simulink model "TrailerSoftware"  (R2019b)
settings: Solver=FixedStepDiscrete  StartTime=0.0  StopTime=inf  FixedStep=update  RelTol=1e-3  EnableMultiTasking=on
values from neighbouring files (symbols this model uses):
  countmax1 = 2500    [ProductionMfile.m]
  countmax2 = 2500    [ProductionMfile.m]
  HeaterIntGain = .0008    (= 0.0008)    [ProductionMfile.m]
  HeatGain = 10    [ProductionMfile.m]
  Intll = 0    [ProductionMfile.m]
  MaxCondPressure = 350    [ProductionMfile.m]
  MinSP = 1    [ProductionMfile.m]
  PostGain100 = 0.0002    [ProductionMfile.m]
  PostGain150 = 0.0005    [ProductionMfile.m]
  PostGain200 = 0.0004    [ProductionMfile.m]
  PostGain300 = 0.0008    [ProductionMfile.m]
  PostInit150 = 12    [ProductionMfile.m]
  PostIntulC = 65    [ProductionMfile.m]
  PostPGain = 0    [ProductionMfile.m]
  PreGain100 = 0.0005    [ProductionMfile.m]
  PreGain150 = 0.0005    [ProductionMfile.m]
  PreGain200 = 0.0003    [ProductionMfile.m]
  PreGain300 = 0.0008    [ProductionMfile.m]
  PreInit150 = 30    [ProductionMfile.m]
  PreIntulC = 65    [ProductionMfile.m]
  PreIntulDH = 65    [ProductionMfile.m]
  PrePGain = 0    [ProductionMfile.m]
  SatPress = [10 20 30 40 50 60 70 80 90 100 110 120 130 140 150 160 170      180 190 200 210 220 230 240 250 260 270 280 290 300 310 320 330      340 350 360 370 380 390 400 410 420 430 440 450 460 470 480 490      500]    [ProductionMfile.m]
  SatTemp = [-29.497 -2.4046 15.401 29.047 40.267 49.88 58.338 65.922 72.819      79.159 85.037 90.526 95.68 100.55 105.16 109.54 113.73 117.73 121.57      125.26 128.82 132.25 135.56 138.77 141.88 144.89 147.82 150.67 153.44      156.15 158.78 161.35 163.85 166.3 168.7 171.04 173.33 175.58 177.77      179.93 182.04 184.11 186.14 188.14 190.09 192.01 193.9 195.75 197.58      199.37]    [ProductionMfile.m]
  SHGain = 2    [ProductionMfile.m]
  SizeCANMatrix = 80    [ProductionMfile.m]
  SizeCOBIDVector = 10    [ProductionMfile.m]
  update = 0.002    [ProductionMfile.m]
undefined symbols (not defined in the file or in its folder): DiscIntNeverNeededParam, PostDGain, PreDGain, Ratio100, Ratio150, Ratio200, Ratio300
libraries: simulink x60, c2837xDlib x35, xpcutilitieslib x24, c2802xlib x8, c280xlib x7, etargetslib x4, svdutilitieslib x2, c2000lib x1
(part 5 of 8)

== stateflow chart TrailerSoftware/SPI Interface/Chart ==
  state Master1
    state Step1
      entry:
      StateNum = 1;
      Ready1 = CheckReady1;
      if GoToMaster == uint16(1);
      GoToTemps= uint16(0);
      else
      GoToTemps = uint16(1);
      end
    state Step2
      entry:
      StateNum = 2;
      if GoToMaster == uint16(1);
      GoToAuxGPIO = uint16(0);
      else
      GoToAuxGPIO = uint16(1);
      end
    state Step3
      entry:
      StateNum = 3;
      if GoToMaster == uint16(1);
      GoToDisplay = uint16(0);
      else
      GoToDisplay = uint16(1);
      end
    state Ready = CheckReady1 [function]
    (default) -> Master1.Step1
    Master1.Step1 -> Master1.Step2 [order 2] : [GoToTemps == uint16(0)]{GoToMaster = uint16(0);}
    Step3 -> Master1.Step1 [order 1] : [GoToDisplay == uint16(0)]{GoToMaster = uint16(0);}
    Master1.Step2 -> Step3 [order 1] : [GoToAuxGPIO == uint16(0)]
        | {GoToMaster = uint16(0);}
  state Display
    state Step1
      entry:
      StateNum = 8;
      GoToMaster = 1;
      DisplayInitComplete = 1;
      GoToDisplay = 0;
    (default) -> Display.Step1
  state AuxGPIO
    state Step1
      entry:
      StateNum = 6;
      GoToAuxGPIO = uint16(0);
      CSLow;
      Write;
      Address(uint16(10)); % Write to ICON
      Data(uint16(8));
      CSHigh
      CSLow;
      Write;
      Address(uint16(0)); % Write to IODIRA
      Data(uint16(0));
      CSHigh
      CSLow;
      Write;
      Address(uint16(1)); % Write to ODIRB
      Data(uint16(255));
      CSHigh
      AuxInitGPIO = uint16(1);
    state CSLow [function]
    state CSHigh [function]
    state Step2
      entry:
      StateNum = 7;
      CSLow;
      Write;
      Address(uint16(18)); % GPIOA Write to outputs
      Data(AuxGPIOOutput);
      CSHigh
      CSLow
      Read;
      Address(uint16(19));  % Read from inputs GPIOB
      AuxGPIOInput = Output;
      CSHigh
      GoToMaster = uint16(1);
    (default) -> AuxGPIO.Step1
    AuxGPIO.Step1 -> AuxGPIO.Step2
  state Temps
    state CSLowTemp1 [function]
    state Step1
      entry:
      StateNum = 4;
      value = uint16(0);
      fault = uint16(0);
      GoToMaster = uint16(0);
      CSLowTemp1;
      Address(uint16(128));
      value = Data(uint16(66));
      CSHighTemp1;
      CSLowTemp1;
      Address(uint16(7));
      fault = Data(uint16(0));
      CSHighTemp1;
      TempsInitComplete = uint16(1);
      GoToMaster = uint16(1);
    state CSHighTemp1 [function]
    state Step2
      entry:
      StateNum = 5;
      GoToMaster = uint16(0);
      CSLowTemp1;
      Address(uint16(1));
      MSB = Data(uint16(0));
      CSHighTemp1;
      CSLowTemp1;
      Address(uint16(2));
      LSB = Data(uint16(0));
      CSHighTemp1;
      [TOut1,TFault1] = TempCal(MSB,LSB);
      GoToMaster = uint16(1);
    state [TOut,TFault] = TempCal(MSB,LSB) [function]
    Temps.Step2 -> (junction 214) : [GoToMaster == uint16(1) ]
    Temps.Step1 -> (junction 214) : [GoToMaster == uint16(1) ]
  state Read [function]
  state Out1 = Data(value) [function]
  state Write [function]
  state Address(value) [function]
  state Contents = Output [function]
  Master1.Step1 -> Temps.Step2 [order 3] : [(GoToTemps == uint16(1) ) &&...
      |   (TempsInitComplete == uint16(1))]
  Master1.Step2 -> AuxGPIO.Step1 [order 3] : [GoToAuxGPIO == uint16(1) && ...
      | AuxInitGPIO == uint16(0)]
  (junction 214) -> Master1.Step1 : [(GoToTemps == uint16(1) ) && ...
      |  (TempsInitComplete == uint16(1))]
  (default) -> Master1
  Master1.Step2 -> AuxGPIO.Step2 [order 2] : [GoToAuxGPIO == uint16(1) && ...
      | AuxInitGPIO == uint16(1)]
  Step3 -> Display.Step1 [order 2] : [GoToDisplay == uint16(1)]
  Master1.Step1 -> Temps.Step1 [order 1] : [(GoToTemps == uint16(1)) &&...
      |  (TempsInitComplete == uint16(0))]
  AuxGPIO.Step2 -> Master1.Step2 : [GoToMaster == uint16(1)]
  Display.Step1 -> Step3 : [GoToMaster == uint16(1)]
  data: Ready function_output size=1; MSB function_input uint16 size=1; LSB function_input uint16 size=1; TOut function_output uint16 size=1; TFault function_output uint16 size=1; value function_input uint16 size=1; Out1 function_output uint16 size=1; value function_input uint16 size=1; Contents function_output uint16; GoToDisplay local uint16 size=1 =uint16(0); GoToAuxGPIO local uint16 size=1 =uint16(0); GoToMaster local uint16 size=1 =uint16(0); GoToTemps local uint16 size=1 =uint16(0); DisplayInitComplete local uint16 size=1 =uint16(0); AuxGPIOOutput input uint16 size=1; AuxGPIOInput output uint16; AuxInitGPIO local; value output; TFault1 output; fault local; TOut1 output; Ready1 local uint16 size=1; StateNum output uint16 size=1; LSB output; MSB output; TempsInitComplete output uint16 size=1 =uint16(0)

== matlab function TrailerSoftware/Subsystem/Display ==
  data: DisRow1 output; DisRow2 output; DisRow3 output; DisRow4 output; StartRow1 output; StartRow2 output; StartRow3 output; StartRow4 output; NumCharRow1 output; NumCharRow2 output; NumCharRow3 output; NumCharRow4 output; ClearDisplay output; DisplayDataAvail output; time input; MBV input; HeaterTempCom input; UseHeater input; CoolTempCom input; PressCommand input; warning1 input; warning2 input; warning3 input; fault1 input; fault2 input; fault3 input; Pulse input; FlowRate input; DuctTemp input; DuctPress input; DuctTempIn input; Hin input; Hout input
function [DisRow1,DisRow2,DisRow3,DisRow4,StartRow1,StartRow2,...
    StartRow3,StartRow4,NumCharRow1,NumCharRow2,NumCharRow3,NumCharRow4,...
    ClearDisplay,DisplayDataAvail]= fcn(time,MBV,...
    HeaterTempCom,UseHeater,CoolTempCom,PressCommand,warning1,warning2,warning3,fault1,fault2,...
    fault3,Pulse,FlowRate,DuctTemp,DuctPress,DuctTempIn,Hin,Hout)
persistent time0 count1 count2 displ  
if isempty(time0)
    time0 = time;
    count1 = 1;
    count2 = 1;
    displ = 0;
end
DisplayDataAvail = 0; %#ok<*NASGU>
if Pulse == 1
    DisplayDataAvail = 1;
end

TempCommand = CoolTempCom;
if UseHeater == 1
    TempCommand = HeaterTempCom;  
end
%#codegen
% MBV(1) = SystemStateValue;
%   Value  Name     Description 
%   0x0090 Menu     Controller is in the menu system
%   0x0093 Off      Controller is in the off mode
%   0x0096 Auto     Controller is in the auto mode
%   0x0099 Failure  Controller is in the failure mode
%   0x009C Running  Controller is in the running mode
% MBV(2) = RunningStateValue;
%   Value  Index        Name               Description
%   0x00   1            No Running         Mode Controller is not in any running state
%   0x01   2            Delay to Start     Controller is delaying to start
%   0x02   3            Preheat            Controller is preheating engine
%   0x03   4            Cranking           Controller is cranking engine
%   0x04   5            Crank Rest         Controller is resting before next crank
%   0x05   6            Crank Success      Controller has successfully started engine
%   0x06   7            Reserved           Reserved
%   0x07   8            Warmup             Controller is warming up engine before applying load
%   0x08   9            Running            Controller is in a normal running state
%   0x09   10           Cooldown           Controller is cooling down engine before shutting down
%   0x0A   11           Shutdown           Controller has shut down the engine
%   0x0B   12           Failure            Controller has shut down the engine due to a fault
%   0x20   13           Remote             Controller was started from 'Start / Stop' switched input
%   0x21   14           Manual             Controller was started from the front panel button
%   0x22   15           Modbus             Controller was started by Modbus command
%   0x23   16           Battery Recharge   Controller was started to recharge batteries
%   0x24   17           Exerciser          Controller was started from the exerciser clock
%   0x25   18           Auxiliary Sensor 1 Controller was started based on Auxiliary Sensor 1 reading
%   0x26   19           Auxiliary Sensor 2 Controller was started based on Auxiliary Sensor 2 reading
%   0x27   20           Loss of Mains      Controller was started due to loss of mains voltage
%   0x28   21           Momentary Switch   Controller was started from 'Momentary' switched input
%   0x29   22           Auxiliary Sensor 3 Controller was started based on Auxiliary Sensor 3 reading
%   0x2A   23           Auxiliary Sensor 4 Controller was started based on Auxiliary Sensor 4 reading
%    RunningState = MBV(2) + 1;


% MBV(3) = EventBitMap1ValueA;
%   Value  Description
%   0      Not In Auto Bit is on due to controller not being in auto mode
%   1      Idle Mode Bit is on due to controller being in idle mode
%   2      Battle Mode Bit is on due to controller being in battle mode
%   3      System OK Bit is on due to controller being free of warnings and failures
%   4      Glowplug Bit is on due to 'Preheat' timer
%   5      Warmup Bit is on due to 'Warmup' timer
%   6      Cooldown Bit is on due to 'Cooldown' timer
%   7      Engine Running Bit is on due to engine running
%   8      Exerciser Bit is on due to engine exercise
%   9      Battery Recharge Bit is on due to battery recharge
%   10     Maintenance Required Bit is on due to 'Maintenance Counter' timer expiring
%   11     Low Battery During Cranking Bit is on due to 'Low Battery Voltage During Cranking'
%   12     N/A
%   13     N/A
%   14     N/A
%   15     N/A 
    
% MBV(4) = EventBitMap1ValueB;
%   0      Delay to Start Bit is on due to 'Delay to Start' timer
%   1      Force Regeneration Bit is on due to a force regeneration (DPF)
%   2      Regeneration Inhibit Bit is on due to regeneration being inhibited (DPF)
%   3 ~ 7  Reserved Reserved
%   8      Fuel Bit is on due to fuel output enabled
%   9      Crank Bit is on due to crank output enabled
%   10     Genset Break1 Bit is on due to transferring to generator position
%   11     Mains Break1 Bit is on due to transferring to mains position
%   12     Pull Coil Bit is on due to pull coil being enabled
%   13     LCD Backlight Bit is on due to the LCD backlight being on
%   14     Voltage Regulator Bit is on when controller is not in idle mode
%   15     Energize to Stop Bit is on due to Energize to Stop timer
% MBV(5) = EventBitMap2ValueA;
%   0      Group Output 1 Bit is on due to output set to Group Output 1 is active
%   1      Group Output 2 Bit is on due to output set to Group Output 2 is active
%   2      Group Output 3 Bit is on due to output set to Group Output 3 is active
%   3      Group Output 4 Bit is on due to output set to Group Output 4 is active
%   4      Increment RPM Bit is on due to the RPM being manually incremented through speed
%          control
%   5      Decrement RPM Bit is on due to the RPM being manually decremented through speed
%          control
%   6      DEF Fluid Pump Bit is on due to DEF Fluid Pump being on
%   7      Genset Disable Bit is on due to the Genset being disabled
%   8      Dummy Load ON Bit is on due to Dummy Load being enabled
%   9 ~ 11 Reserved Reserved
%   12     Glowplug Bit is on due to preheat input or ECM preheat being active
%   13     Common Fault Bit is on due to a any fault occurring
%   14     Temperature Unit Reserved - Fixed to Fahrenheit
%   15     Pressure Unit Reserved - Fixed to PSI
% MBV(6) = EventBitMap2ValueB;
%   0      Overcrank Warning Bit is on due to controller failing to crank engine on first attempt
%   1      Invalid Setting Warning Bit is on due to an invalid setting being stored in the controller
%   2      Emergency Input Bit is on due to Emergency Stop input being active
%   3      EPS Load is On Bit is on due to current readings being at least 5% of the rated current
%          setting
%   4      Genset Break On1 Reserved
%   5      Mains Break On1 Reserved
%   6      Mains Pickup1 Bit is on due to mains voltage being within acceptable levels after
%          dropping out
%   7      Mains Dropout1 Bit is on due to controller sensing mains voltage has dropped out
%   8      Mains OK1 Bit is on due to mains voltage being within acceptable levels
%   9      Start Inhibit Bit is on due to Start Inhibit input being active
%   10     Remote Reset Bit is on due to the Remote Reset input being active
%   11 ~15 N/A
% MBV(7) = FaultBitMapValueA;
%   Bit   Name                  Description
%   0     Overcrank             Fault due to max attempts at cranking
%   without starting (1)
%   1     Engine Failed to Stop Fault due to engine speed not being 0 RPM
%   at shutdown (2)
%   2     DM1 Stop Lamp1        DM1 Stop Lamp is on (not used) (3)
%   3     High Engine Temp      Fault due to high engine temperature (4)
%   4     Low Oil Pressure      Fault due to low oil pressure (5)
%   5     Low Fuel Level        Fault due to low fuel level (6)
%   6     Under Speed           Fault due to low engine speed (7)
%   7     Over Speed            Fault due to high engine speed (8)
%   8     Low Battery Voltage   Fault due to low battery voltage (9)
%   9     High Battery Voltage  Fault due to high battery voltage (10)
%   10    Low Coolant Level     Fault due to low coolant level (11)
%   11    Low Air Pressure      Fault due to low air pressure (not used)
%   (12)
%   12    Low Hydraulic Press   Fault due to low hydraulic pressure (not
%   used) (13)
%   13    Under Frequency       Fault due to low AC frequency (14)
%   14    Over Frequency        Fault due to high AC frequency (15)
%   15    AC Under Voltage      Fault due to low AC voltage (16)
% MBV(8) = FaultBitMapValueB;
%   0     AC Over Voltage       Fault due to high AC voltage (17)
%   1     ECM Communication     Fault due to loss of communications with
%   ECM (18)
%   2     Configurable Failure 1 Fault due to Configurable Fail Input 1
%   being active (not used) (19)
%   3     Configurable Failure 2 Fault due to Configurable Fail Input 2
%   being active (not used) (20)
%   4     Auxiliary Sensor 1    Fault due to low / high reading on
%   Auxiliary Sensor 1  (not used) (21)
%   5     Auxiliary Sensor 2    Fault due to low / high reading on
%   Auxiliary Sensor 2 (not used) (22)
%   6     Auxiliary Sensor 3    Fault due to low / high reading on Auxiliary Sensor 3 
%   (not used) (23)
%   7     Auxiliary Sensor 4    Fault due to low / high reading on
%   Auxiliary Sensor 4 (not used) (24)
%   8     Over Current          Fault due to high current reading (25)
%   9     Configurable Failure 3 Fault due to Configurable Fail Input 3
%   being active (not used) (26)
%   26 ~ 31 Reserved Reserved (not used) (27-32)
       
%   Bit   Name                  Description
%   0     Low Engine Temp       Warning due to low engine temperature
%   1     High Engine Temp      Warning due to high engine temperature
%   2     Low Oil Pressure      Warning due to low oil pressure
%   3     Under Speed           Warning due to low engine speed
%   4     Over Speed            Warning due to high engine speed
%   5     Low Fuel Level        Warning due to low fuel level
%   6     High Fuel Level       Warning due to high fuel level
%   7     Low Battery Voltage   Warning due to low battery voltage
%   8     High Battery Voltage  Warning due to high battery voltage
%   9     Under Frequency       Warning due to low AC frequency
%   10    Over Frequency        Warning due to high AC frequency
%   11    AC Under Voltage      Warning due to low AC voltage
%   12    AC Over Voltage       Warning due to high AC voltage
%   13    Battery Charger Fault Warning due to battery charger fault
%   14    Over Current          Warning due to high AC current
%   15    Fuel In Basin         Warning due to fuel being in the catch basin
% MBV(10) = WarningBitMapValueB;
%   Bit   Name                  Description
%   0     Configurable Warning 1 Warning due to Configurable Warn Input 1 being active
%   1     Configurable Warning 2 Warning due to Configurable Warn Input 2 being active
%   2     Auxiliary Sensor 1     Warning due to low / high reading on Auxiliary Sensor 1
%   3     Auxiliary Sensor 2     Warning due to low / high reading on Auxiliary Sensor 2
%   4     Auxiliary Sensor 3     Warning due to low / high reading on Auxiliary Sensor 3
%   5     Auxiliary Sensor 4     Warning due to low / high reading on Auxiliary Sensor 4
%   6 ~ 15 Reserved Reserved
% MBV(11) = GenFreqValue;
% MBV(12) = GenVoltValueA;
% MBV(13) = GenVoltValueB;
% MBV(14) = GenVoltValueC;
% MBV(15) = GenCurValueA;
% MBV(16) = GenCurValueB;
% MBV(17) = GenCurValueC;
% MBV(18) = EngineTempValue;
% MBV(19) = EngineOilPressValue;
% MBV(20) = FuelLevelValue;
% MBV(21) = BatteryVoltValue;
% MBV(22) = EngineRunHoursValue;
% MBV(23) = FCSuperHeatValue;
% MBV(24) = RCSuperHeatValue;
% MBV(25) = SuctionPressValue;
% MBV(26) = FSatTempValue;
% MBV(27) = RSatTempValue;
% MBV(28) = FSucTempValue;
% MBV(29) = RSucTempValue;
% MBV(30) = FRmTempValue;
% MBV(31) = RRmTempValue;
% MBV(32) = FValPosValue;
% MBV(33) = RValPosValue;
% MBV(34) = FEvapTempValue;
% MBV(35) = REvapTempValue;
% MBV(36) = FAlarmValue;
% MBV(37) = RAlarmValue;

FuelLevelValue = MBV(20);
s1 = convertnum(FuelLevelValue);
s2 = convertnum(FlowRate);
s6 = convertnum(min(140,max(TempCommand,0)));
s7 = convertnum(min(9,max(PressCommand,0)));
s8 = convertnum(min(140,max(DuctTemp,0)));
s9 = convertnum(min(9,max(DuctPress,0)));
s10 = convertnum(min(140,max(DuctTempIn,0)));
s11 = convertnum(min(99,max(Hin,0)));
s12 = convertnum(min(99,max(Hout,0)));
Message1 = ['TempSet ' s6(1:3)...
    ',Meas' s8(1:3) 'F'];
Message2 = ['PSet' s7(1:4)...
    ',Meas' s9(1:4) 'psi'];
Message3 = ['Inlet Air Temp: ' s10...
    ', deg F  ','Fuel Level ' s1...
    ',% ' 'Humidity Inlet ' s11...
    ',% ' 'Humidity Outlet ' s12...
    ',% '  'Flow Rate Selected = ' s2...
    ', lbm/min'];
    
s4A = convertnum(min(999,max(warning1,0)));
s4B = convertnum(min(999,max(warning2,0)));
s4C = convertnum(min(999,max(warning3,0)));
s5A = convertnum(min(999,max(fault1,0)));
s5B = convertnum(min(999,max(fault2,0)));
s5C = convertnum(min(999,max(fault3,0)));

 Message4 = [' Warning = ' s4A ' ' s4B ' ' s4C ' Fault = ' s5A...
        ' ' s5B ' ' s5C ' '];

DisRow1 = uint8(32*ones(20,1));
DisRow2 = uint8(32*ones(20,1));
DisRow3 = uint8(32*ones(20,1));
DisRow4 = uint8(32*ones(20,1));
StartRow1 = uint8(1);
StartRow2 = uint8(1);
StartRow3 = uint8(1);
StartRow4 = uint8(1);
NumCharRow1 = uint8(20);
NumCharRow2 = uint8(20);
NumCharRow3 = uint8(20);
NumCharRow4 = uint8(20);
ClearDisplay = uint8(0);
DisplayDataAvail = uint8(0);
if displ == 1
    DisplayDataAvail = uint8(1);
    displ = 0;
end
if time > time0 + .5
    time0 = time;
    displ = 1;
    count1 = count1 + 1;
    count2 = count2 + 1;
    if count1 == length(Message3) - 20
        count1 = 1;
    end
    if count2 == length(Message4) - 20
        count2 = 1;
    end
end
    
DisRow1(:,1) = Message1;
DisRow2(:,1) = Message2;
DisRow3(:,1) = Message3(1,count1:count1+19)';
DisRow4(:,1) = Message4(1,count2:count2+19)';

return

% Convert number to string
function y = convertnum(input)
    y = uint8(32*ones(1,5));
    int_part = double(floor(input));
    float_part = input - double(int_part);
    i = 1;
    temp = int_part;
    if temp < 10
        y(i) = uint8(temp + 48);  
        i = 2;
    elseif floor(temp/10) < 10
        y(i) = uint8(floor(temp/10)+48);
        y(i+1) = uint8((temp - floor(temp/10)*10) + 48);
        i = 3;
    elseif floor(temp/100) < 10
        y(i) = uint8(floor(temp/100)+48);
        y(i+1) = uint8(floor((temp - floor(temp/100)*100)/10) + 48);
        y(i+2) = uint8((temp - floor(temp/10)*10) + 48);
        i = 4;
    end
    y(i) = '.';
    temp = float_part;
    i = i + 1;
    if temp*10 < 10
        y(i) = uint8((temp*10) + 48);  
    end
    
return

== matlab function TrailerSoftware/Subsystem/Modbus Routine ==
  data: ModbusInputReady input uint8; ModbusOutReady output uint8; ModbusInputVector input; ModbusOutVector output size=[1,8]; time input; ModbusVector output size=39; countoutputout output; ManualMode2StatusOut output size=1; ManualMode3StatusOut output size=1; Failcountout output; Goodcountout output; FaultBitMapValueAOut output
function [ModbusOutReady,ModbusOutVector,ModbusVector,...
    countoutputout,ManualMode2StatusOut,...
    ManualMode3StatusOut,Failcountout,Goodcountout,...
    FaultBitMapValueAOut] = fcn1(ModbusInputReady,ModbusInputVector,time)
persistent SystemState RunningState EventBitMap1A EventBitMap1B ...
    EventBitMap2A EventBitMap2B FaultBitMapA FaultBitMapB WarningBitMapA ...
    WarningBitMapB GenFreq GenVoltA GenVoltB GenVoltC GenCurA GenCurB ...
    GenCurC EngineTemp EngineOilPress FuelLevel EngineRunHours....
    BatteryVolt State time0 SystemStateValue ...
    RunningStateValue EventBitMap1ValueA  EventBitMap1ValueB ...
    EventBitMap2ValueA EventBitMap2ValueB FaultBitMapValueA ...
    FaultBitMapValueB WarningBitMapValueA WarningBitMapValueB ...
    GenFreqValue GenVoltValueA GenVoltValueB GenVoltValueC ...
    GenCurValueA GenCurValueB GenCurValueC EngineTempValue ...
    EngineOilPressValue FuelLevelValue BatteryVoltValue ...
    EngineRunHoursValue  countinput...
    countoutput ManualMode2Status...
    ManualMode3Status complete Failcount Goodcount SuctionOutCnt...
    SuctionInCnt Goodcount1300
if isempty(SystemState)
    
    SystemState = [hex2dec('01') hex2dec('03') hex2dec('00')...
                hex2dec('A7') hex2dec('00') hex2dec('01')...
                hex2dec('35') hex2dec('E9')];
    RunningState = [hex2dec('01') hex2dec('03') hex2dec('00')...
                hex2dec('A8') hex2dec('00') hex2dec('01')...
                hex2dec('05') hex2dec('EA')];
    EventBitMap1A = [hex2dec('01') hex2dec('03') hex2dec('00')...
                hex2dec('B6') hex2dec('00') hex2dec('01')...
                hex2dec('65') hex2dec('EC')];
    EventBitMap1B = [hex2dec('01') hex2dec('03') hex2dec('00')...
                hex2dec('B7') hex2dec('00') hex2dec('01')...
                hex2dec('34') hex2dec('2C')];    
    EventBitMap2A = [hex2dec('01') hex2dec('03') hex2dec('00')...
                hex2dec('B8') hex2dec('00') hex2dec('01')...
                hex2dec('04') hex2dec('2F')];
    EventBitMap2B = [hex2dec('01') hex2dec('03') hex2dec('00')...
                hex2dec('B7') hex2dec('00') hex2dec('01')...
                hex2dec('34') hex2dec('2C')];
    FaultBitMapA = [hex2dec('01') hex2dec('03') hex2dec('00')...
                hex2dec('B5') hex2dec('00') hex2dec('01')...
                hex2dec('95') hex2dec('EC')];
    FaultBitMapB = [hex2dec('01') hex2dec('03') hex2dec('00')...
                hex2dec('B6') hex2dec('00') hex2dec('01')...
                hex2dec('65') hex2dec('EC')];
    WarningBitMapA = [hex2dec('01') hex2dec('03') hex2dec('00')...
                hex2dec('B2') hex2dec('00') hex2dec('01')...
                hex2dec('24') hex2dec('2D')];
    WarningBitMapB = [hex2dec('01') hex2dec('03') hex2dec('00')...
                hex2dec('B3') hex2dec('00') hex2dec('01')...
                hex2dec('75') hex2dec('ED')];
    GenFreq = [hex2dec('01') hex2dec('03') hex2dec('00')...
                hex2dec('99') hex2dec('00') hex2dec('01')...
                hex2dec('54') hex2dec('25')];
    GenVoltA = [hex2dec('01') hex2dec('03') hex2dec('00')...
                hex2dec('9B') hex2dec('00') hex2dec('01')...
                hex2dec('F5') hex2dec('E5')];
    GenVoltB = [hex2dec('01') hex2dec('03') hex2dec('00')...
                hex2dec('9C') hex2dec('00') hex2dec('01')...
                hex2dec('44') hex2dec('24')];
    GenVoltC = [hex2dec('01') hex2dec('03') hex2dec('00')...
                hex2dec('9D') hex2dec('00') hex2dec('01')...
                hex2dec('15') hex2dec('E4')];
    GenCurA = [hex2dec('01') hex2dec('03') hex2dec('00')...
                hex2dec('9E') hex2dec('00') hex2dec('01')...
                hex2dec('E5') hex2dec('E4')];
    GenCurB = [hex2dec('01') hex2dec('03') hex2dec('00')...
                hex2dec('9F') hex2dec('00') hex2dec('01')...
                hex2dec('B4') hex2dec('24')];
    GenCurC = [hex2dec('01') hex2dec('03') hex2dec('00')...
                hex2dec('A0') hex2dec('00') hex2dec('01')...
                hex2dec('84') hex2dec('28')];
    EngineTemp = [hex2dec('01') hex2dec('03') hex2dec('00')...
                hex2dec('96') hex2dec('00') hex2dec('01')...
                hex2dec('64') hex2dec('26')];
    EngineOilPress = [hex2dec('01') hex2dec('03') hex2dec('00')...
                hex2dec('97') hex2dec('00') hex2dec('01')...
                hex2dec('35') hex2dec('E6')];
    FuelLevel = [hex2dec('01') hex2dec('03') hex2dec('00')...
                hex2dec('98') hex2dec('00') hex2dec('01')...
                hex2dec('05') hex2dec('E5')];
    BatteryVolt = [hex2dec('01') hex2dec('03') hex2dec('00')...
                hex2dec('9A') hex2dec('00') hex2dec('01')...
                hex2dec('A4') hex2dec('25')];
    EngineRunHours = [hex2dec('01') hex2dec('03') hex2dec('00')...
                hex2dec('A3') hex2dec('00') hex2dec('01')...
                hex2dec('74') hex2dec('28')];
    Goodcount1300 = 0;        
    State = 0;
    time0 = time;
    SystemStateValue = 0;
    RunningStateValue = 0;
    EventBitMap1ValueA = 0;
    EventBitMap1ValueB = 0;
    EventBitMap2ValueA = 0;
    EventBitMap2ValueB = 0;
    FaultBitMapValueA = 0;
    FaultBitMapValueB = 0;
    WarningBitMapValueA = 0;
    WarningBitMapValueB = 0;
    GenFreqValue = 0;
    GenVoltValueA = 0;
    GenVoltValueB = 0;
    GenVoltValueC = 0;
    GenCurValueA = 0;
    GenCurValueB = 0;
    GenCurValueC = 0;
    EngineTempValue = 0;
    EngineOilPressValue = 0;
    FuelLevelValue = 0;
    BatteryVoltValue = 0;
    EngineRunHoursValue = 0;
    countinput = 0;
    countoutput = 0;
    ManualMode2Status = 0;
    ManualMode3Status = 0;
    complete = 1;
    Failcount = 0;
    Goodcount = 0;
    SuctionOutCnt = 0;
    SuctionInCnt = 0;
end
%#codegen
if ModbusInputReady == 1
    countinput = countinput + 1;
end
countinputout = countinput;
ModbusOutReady = 0;
ModbusOutVector = SystemState;
%waittime1 = .75;
%waittime2 = 1.5;
%waittime3 = .01;
%waittime4 = .01;
timeout = 2;
ModbusVector = zeros(39,1);
countoutputout =  countoutput;
ManualMode2StatusOut = uint8(ManualMode2Status);
ManualMode3StatusOut = uint8(ManualMode3Status);
AutoMode =  double(not((bitget(uint32(EventBitMap1ValueA),1))));
Failcountout = Failcount;
Goodcountout = Goodcount;
SuctionOutCntOut = SuctionOutCnt;
SuctionInCntOut = SuctionInCnt;
Goodcount1300Out = Goodcount1300;
FaultBitMapValueAOut=FaultBitMapValueA;
switch State
    case 0
        ModbusOutVector = SystemState;
        ModbusOutReady = 1;
        State = 100;
        time0 = time;
    case 100
       if complete == 1
            State = 200;
            complete = 0;
       end
       if (time-time0) > timeout
            State = 200;
            complete = 0;
            Failcount = Failcount + 1;
       end 
    case 200
        ModbusOutVector = RunningState;
        ModbusOutReady = 1;
        State = 300;
        time0 = time;
    case 300
        if complete == 1
            State = 400;
            complete = 0;
        end
        if (time-time0) > timeout
            State = 400;
            complete = 0;
            Failcount = Failcount + 1;
       end 
    case 400
        ModbusOutVector = EventBitMap1A;
        ModbusOutReady = 1;
        State = 500;
        time0 = time;
    case 500
        if complete == 1
            State = 600;
            complete = 0;
        end
        if (time-time0) > timeout
            State = 600;
            complete = 0;
            Failcount = Failcount + 1;
       end 
    case 600
        ModbusOutVector = EventBitMap1B;
        ModbusOutReady = 1;
        State = 700;
        time0 = time;
    case 700
        if complete == 1
            State = 800;
            complete = 0;
        end
        if (time-time0) > timeout
            State = 800;
            complete = 0;
            Failcount = Failcount + 1;
        end 
    case 800
        ModbusOutVector = EventBitMap2A;
        ModbusOutReady = 1;
        State = 900;
        time0 = time;
    case 900
        if complete == 1
            State = 1000;
            complete = 0;
        end
        if (time-time0) > timeout
            State = 1000;
            complete = 0;
            Failcount = Failcount + 1;
       end 
    case 1000
        ModbusOutVector = EventBitMap2B;
        ModbusOutReady = 1;
        State = 1100;
        time0 = time;
    case 1100
        if complete == 1
            State = 1200;
            complete = 0;
        end
        if (time-time0) > timeout
            State = 1200;
            complete = 0;
            Failcount = Failcount + 1;
       end 
    case 1200
        ModbusOutVector = FaultBitMapA;
        ModbusOutReady = 1;
        State = 1300;
        time0 = time;
    case 1300
        if complete == 1
            State = 1400;
            complete = 0;
        end
        if (time-time0) > timeout
            State = 1400;
            complete = 0;
            Failcount = Failcount + 1;
       end 
    case 1400
        ModbusOutVector = FaultBitMapB;
        ModbusOutReady = 1;
        State = 1500;
        time0 = time;
    case 1500
        if complete == 1
            State = 1600;
            complete = 0;
        end
        if (time-time0) > timeout
            State = 1600;
            complete = 0;
            Failcount = Failcount + 1;
       end 
    case 1600
        ModbusOutVector = WarningBitMapA;
        ModbusOutReady = 1;
        State = 1700;
        time0 = time;
    case 1700
        if complete == 1
            State = 1800;
            complete = 0;
        end
        if (time-time0) > timeout
            State = 1800;
            complete = 0;
            Failcount = Failcount + 1;
       end 
    case 1800
        ModbusOutVector = WarningBitMapB;
        ModbusOutReady = 1;
        State = 1900;
        time0 = time;
    case 1900
        if complete == 1
            State = 2000;
            complete = 0;
        end
        if (time-time0) > timeout
            State = 2000;
            complete = 0;
            Failcount = Failcount + 1;
       end 
    case 2000
        ModbusOutVector = GenFreq;
        ModbusOutReady = 1;
        State = 2100;
        time0 = time;
    case 2100
         if complete == 1
            State = 2200;
            complete = 0;
        end
        if (time-time0) > timeout
            State = 2200;
            complete = 0;
            Failcount = Failcount + 1;
       end 
    case 2200
        ModbusOutVector = GenVoltA;
        ModbusOutReady = 1;
        State = 2300;
        time0 = time;
    case 2300
        if complete == 1
            State = 2400;
            complete = 0;
        end
        if (time-time0) > timeout
            State = 2400;
            complete = 0;
            Failcount = Failcount + 1;
       end 
    case 2400
        ModbusOutVector = GenVoltB;
        ModbusOutReady = 1;
        State = 2500;
        time0 = time;
    case 2500
        if complete == 1
            State = 2600;
            complete = 0;
        end
        if (time-time0) > timeout
            State = 2600;
            complete = 0;
            Failcount = Failcount + 1;
       end 
    case 2600
        ModbusOutVector = GenVoltC;
        ModbusOutReady = 1;
        State = 2700;
        time0 = time;
    case 2700
        if complete == 1
            State = 2800;
            complete = 0;
        end
        if (time-time0) > timeout
            State = 2800;
            complete = 0;
            Failcount = Failcount + 1;
       end 
    case 2800
        ModbusOutVector = GenCurA;
        ModbusOutReady = 1;
        State = 2900;
        time0 = time;
    case 2900
        if complete == 1
            State = 3000;
            complete = 0;
        end
        if (time-time0) > timeout
            State = 3000;
            complete = 0;
            Failcount = Failcount + 1;
       end 
    case 3000
        ModbusOutVector = GenCurB;
        ModbusOutReady = 1;
        State = 3100;
        time0 = time;
    case 3100
        if complete == 1
            State = 3200;
            complete = 0;
        end
        if (time-time0) > timeout
            State = 3200;
            complete = 0;
            Failcount = Failcount + 1;
       end 
    case 3200
        ModbusOutVector = GenCurC;
        ModbusOutReady = 1;
        State = 3300;
        time0 = time;
    case 3300   
        if complete == 1
            State = 3400;
            complete = 0;
        end
        if (time-time0) > timeout
            State = 3400;
            complete = 0;
            Failcount = Failcount + 1;
       end 
    case 3400
        ModbusOutVector = EngineTemp;
        ModbusOutReady = 1;
        State = 3500;
        time0 = time;
    case 3500
        if complete == 1
            State = 3600;
            complete = 0;
        end
        if (time-time0) > timeout
            State = 3600;
            complete = 0;
            Failcount = Failcount + 1;
       end 
    case 3600
        ModbusOutVector = EngineOilPress;
        ModbusOutReady = 1;
        State = 3700;
        time0 = time;
    case 3700
        if complete == 1
            State = 3800;
            complete = 0;
        end
        if (time-time0) > timeout
            State = 3800;
            complete = 0;
            Failcount = Failcount + 1;
       end 
    case 3800
        ModbusOutVector = FuelLevel;
        ModbusOutReady = 1;
        State = 3900;
        time0 = time;
    case 3900
        if complete == 1
            State = 4000;
            complete = 0;
        end
        if (time-time0) > timeout
            State = 4000;
            complete = 0;
            Failcount = Failcount + 1;
       end 
    case 4000
        ModbusOutVector = BatteryVolt;
        ModbusOutReady = 1;
        State = 4100;
        time0 = time;
    case 4100
        if complete == 1
            State = 4200;
            complete = 0;
        end
        if (time-time0) > timeout
            State = 4200;
            complete = 0;
            Failcount = Failcount + 1;
       end 
    case 4200
        ModbusOutVector = EngineRunHours;
        ModbusOutReady = 1;
        State = 4300;
        time0 = time;
    case 4300
        if complete == 1
            State = 0;
            complete = 0;
        end
        if (time-time0) > timeout
            State = 0;
            complete = 0;
           Failcount = Failcount + 1;
        end 
end
    
Fail = 0; %#ok<NASGU>
              
if ModbusInputReady == 1
    if (State == 100  && complete == 0)
       [SystemStateValuet,Fail] = ReadValue(ModbusInputVector,7);
        complete = 1;
       if Fail ~= 1
          SystemStateValue = SystemStateValuet;
        %  Goodcount = Goodcount + 1;
       else
           %Failcount = Failcount + 1;
       end
    end
    if (State == 300 && complete == 0)
        [RunningStateValuet,Fail] = ReadValue(ModbusInputVector,7);
        complete = 1;
        if Fail ~= 1
           RunningStateValue = RunningStateValuet; 
         %  Goodcount = Goodcount + 1;
       else
           %Failcount = Failcount + 1;
       end
    end
    if (State == 500 && complete == 0)
        [EventBitMap1ValueAt,Fail] = ReadValue(ModbusInputVector,7);
        complete = 1;
        if Fail ~= 1
            EventBitMap1ValueA = EventBitMap1ValueAt;
           % Goodcount = Goodcount + 1;
       else
           %Failcount = Failcount + 1;
       end
    end
    if (State == 700 && complete == 0)
        [EventBitMap1ValueBt,Fail] = ReadValue(ModbusInputVector,7);
        complete = 1;
        if Fail ~= 1
            EventBitMap1ValueB = EventBitMap1ValueBt;
          %  Goodcount = Goodcount + 1;
       else
           %Failcount = Failcount + 1;
       end
    end
    if (State == 900 && complete == 0)
        [EventBitMap2ValueAt,Fail] = ReadValue(ModbusInputVector,7);
        complete = 1;
        if Fail ~= 1
            EventBitMap2ValueA = EventBitMap2ValueAt;
        %    Goodcount = Goodcount + 1;
       else
           %Failcount = Failcount + 1;
       end
    end
    if (State == 1100 && complete == 0)
        [EventBitMap2ValueBt,Fail] = ReadValue(ModbusInputVector,7);
        complete = 1;
        if Fail ~= 1
            EventBitMap2ValueB = EventBitMap2ValueBt;
          %  Goodcount = Goodcount + 1;
        else
           %Failcount = Failcount + 1;
       end            
    end
    if (State == 1300)
        [FaultBitMapValueAt,Fail] = ReadValue(ModbusInputVector,7);
        if Fail ~= 1
            FaultBitMapValueA = FaultBitMapValueAt;
           % Goodcount = Goodcount + 1;
            complete = 1;
       else
           %Failcount = Failcount + 1;
       end
    end
    if (State == 1500)
        [FaultBitMapValueBt,Fail] = ReadValue(ModbusInputVector,7);
        if Fail ~= 1
            FaultBitMapValueB = FaultBitMapValueBt;
           % Goodcount = Goodcount + 1;
            complete = 1;
       else
           %Failcount = Failcount + 1;
       end           
    end
    if (State == 1700)
        [WarningBitMapValueAt,Fail] = ReadValue(ModbusInputVector,7);
        if Fail ~= 1
            WarningBitMapValueA = WarningBitMapValueAt;
            %Goodcount = Goodcount + 1;
            complete = 1;
       else
           %Failcount = Failcount + 1;
       end
    end
    if (State == 1900)
        [WarningBitMapValueBt,Fail] = ReadValue(ModbusInputVector,7);
        if Fail ~= 1
            WarningBitMapValueB = WarningBitMapValueBt;
           % Goodcount = Goodcount + 1;
            complete = 1;
       else
           %Failcount = Failcount + 1;
       end            
    end
    if (State == 2100)
        [GenFreqValuet,Fail] = ReadValue(ModbusInputVector,7);
        if Fail ~= 1
            GenFreqValue = GenFreqValuet/10;
           % Goodcount = Goodcount + 1;
            complete = 1;
        end
    end
    if (State == 2300)
        [GenVoltValueAt,Fail] = ReadValue(ModbusInputVector,7);
        if Fail ~= 1
            GenVoltValueA = GenVoltValueAt/10;
           % Goodcount = Goodcount + 1;
            complete = 1;
       else
           %Failcount = Failcount + 1;
       end            
    end
    if (State == 2500)
        [GenVoltValueBt,Fail] = ReadValue(ModbusInputVector,7);
        if Fail ~= 1
            GenVoltValueB = GenVoltValueBt/10;
           % Goodcount = Goodcount + 1;
            complete = 1;
       else
           %Failcount = Failcount + 1;
       end              
    end
    if (State == 2700)
        [GenVoltValueCt,Fail] = ReadValue(ModbusInputVector,7);
        if Fail ~= 1
            GenVoltValueC = GenVoltValueCt/10;
         %   Goodcount = Goodcount + 1;
            complete = 1;
       else
           %Failcount = Failcount + 1;
       end
    end
    if (State == 2900)
        [GenCurValueAt,Fail] = ReadValue(ModbusInputVector,7);
        if Fail ~= 1
            GenCurValueA = GenCurValueAt/10;
         %   Goodcount = Goodcount + 1;
            complete = 1;
       else
           %Failcount = Failcount + 1;
       end
    end
    if (State == 3100)
        [GenCurValueBt,Fail] = ReadValue(ModbusInputVector,7);
        if Fail ~= 1
            GenCurValueB = GenCurValueBt/10;
            complete = 1;
          %  Goodcount = Goodcount + 1;
       else
           %Failcount = Failcount + 1;
       end
    end
    if (State == 3300)
        [GenCurValueCt,Fail] = ReadValue(ModbusInputVector,7);
        if Fail ~= 1
            GenCurValueC = GenCurValueCt/10;
            complete = 1;
          %  Goodcount = Goodcount + 1;
       else
           %Failcount = Failcount + 1;
       end            
    end 
    if (State == 3500)
        [EngineTempValuet,Fail] = ReadValue(ModbusInputVector,7);
        if Fail ~= 1
            EngineTempValue = EngineTempValuet/10;
            complete = 1;
          %  Goodcount = Goodcount + 1;
       else
           %Failcount = Failcount + 1;
       end             
    end 
    if (State == 3700)
        [EngineOilPressValuet,Fail] = ReadValue(ModbusInputVector,7);
        if Fail ~= 1
            EngineOilPressValue = EngineOilPressValuet/10;
            complete = 1;
          %  Goodcount = Goodcount + 1;
       else
           %Failcount = Failcount + 1;
       end            
    end 
    if (State == 3900)
        [FuelLevelValuet,Fail] = ReadValue(ModbusInputVector,7);
        if Fail ~= 1
            FuelLevelValue = FuelLevelValuet/10;
            complete = 1;
            %Goodcount = Goodcount + 1;
       else
           %Failcount = Failcount + 1;
       end        
    end 
    if (State == 4100)
        [BatteryVoltValuet,Fail] = ReadValue(ModbusInputVector,7);
        if Fail ~= 1
            BatteryVoltValue = BatteryVoltValuet/10;
            complete = 1;
           % Goodcount = Goodcount + 1;
       else
          % Failcount = Failcount + 1;
       end
    end 
    if (State == 4300)
        [EngineRunHoursValuet,Fail] = ReadValue(ModbusInputVector,7);
        if Fail ~= 1
           EngineRunHoursValue = EngineRunHoursValuet/10;
            complete = 1;
           % Goodcount = Goodcount + 1;
       else
           %Failcount = Failcount + 1;
       end
    end 
    
end


StateOut = State;
ModbusVector(1,1) = SystemStateValue;
ModbusVector(2,1) = RunningStateValue;
ModbusVector(3,1) = EventBitMap1ValueA;
ModbusVector(4,1) = EventBitMap1ValueB;
ModbusVector(5,1) = EventBitMap2ValueA;
ModbusVector(6,1) = EventBitMap2ValueB;
ModbusVector(7,1) = FaultBitMapValueA;
ModbusVector(8,1) = FaultBitMapValueB;
ModbusVector(9,1) = WarningBitMapValueA;
ModbusVector(10,1) = WarningBitMapValueB;
ModbusVector(11,1) = GenFreqValue;
ModbusVector(12,1) = GenVoltValueA;
ModbusVector(13,1) = GenVoltValueB;
ModbusVector(14,1) = GenVoltValueC;
ModbusVector(15,1) = GenCurValueA;
ModbusVector(16,1) = GenCurValueB;
ModbusVector(17,1) = GenCurValueC;
ModbusVector(18,1) = EngineTempValue;
ModbusVector(19,1) = EngineOilPressValue;
ModbusVector(20,1) = FuelLevelValue;
ModbusVector(21,1) = BatteryVoltValue;
ModbusVector(22,1) = EngineRunHoursValue;

if ModbusOutReady == 1
    countoutput = countoutput + 1;
end

return

function [Value,Fail] = ReadValue(ModbusInputVector,N)
    crcreg = uint16(hex2dec('FFFF'));
    GENPOLY = hex2dec('A001'); 
    Value = 0;
    for i = 1:N-2
        crcreg = bitxor(crcreg,uint16(ModbusInputVector(i)));
        for j = 1:8
            if bitand(crcreg,1)
                crcreg = bitshift(crcreg,-1);
                crcreg = bitxor(crcreg,GENPOLY);
            else
                crcreg = bitshift(crcreg,-1);
            end
        end
    end
    Fail = 0;
    CRC = uint16(bitor(bitshift(uint16(ModbusInputVector(N)),...
        8),uint16(ModbusInputVector(N-1))));
    if CRC == crcreg
        if N == 6
            Value = double(uint16(ModbusInputVector(N-2)));
        else
            Value = double(bitor(bitshift(uint16...
                (ModbusInputVector(N-3)),8),uint16(ModbusInputVector(N-2))));
        end
    else
        Fail = 1;
    end
return
